simulink model "exampleModel_bus_axi_w_4ptavg"  (R2017b)
settings: Solver=VariableStepAuto  StartTime=0.0  StopTime=10e-5  RelTol=1e-3
PreLoadFcn:
  | setup
values from neighbouring files (symbols this model uses):
  axiClk = 156.25e6    (= 156250000)    [setup.m]    (also in setup_exampleModel_bus_axi_simulink.m; setup_exampleModel_bus_axi_simulink_lcls2.m; setup_lcls2_pcav.m; sysgen_signal.m)
  cav1p1_addr = 204    [setup_exampleModel_bus_axi_simulink.m]    (also in setup_exampleModel_bus_axi_simulink_lcls2.m; setup_lcls2_pcav.m; sysgen_signal.m)
  cav1p2_addr = cav1p1_addr * 2    (= 408)    [setup_exampleModel_bus_axi_simulink.m]    (also in setup_exampleModel_bus_axi_simulink_lcls2.m; setup_lcls2_pcav.m; sysgen_signal.m)
  cav2p1_addr = cav1p1_addr * 3    (= 612)    [setup_exampleModel_bus_axi_simulink.m]    (also in setup_exampleModel_bus_axi_simulink_lcls2.m; setup_lcls2_pcav.m; sysgen_signal.m)
  cav2p2_addr = cav1p1_addr * 4    (= 816)    [setup_exampleModel_bus_axi_simulink.m]    (also in setup_exampleModel_bus_axi_simulink_lcls2.m; setup_lcls2_pcav.m; sysgen_signal.m)
  Fadc = Fs/interleavedChannels    (= 29750000)    [setup.m]    (also in setup_exampleModel_bus_axi_simulink.m = 357000000; setup_exampleModel_bus_axi_simulink_lcls2.m = 351000000; setup_lcls2_pcav.m = 357000000; sysgen_signal.m = 357000000)
  fir_lpf = fir1(15, w_lpf)    [setup_exampleModel_bus_axi_simulink.m]    (also in setup_exampleModel_bus_axi_simulink_lcls2.m; setup_lcls2_pcav.m)
  Fproc = 204e6    (= 204000000)    [setup_exampleModel_bus_axi_simulink.m]    (also in setup_exampleModel_bus_axi_simulink_lcls2.m = 200571400; setup_lcls2_pcav.m; sysgen_signal.m)
  Fsig = Fproc/12    (= 17000000)    [setup_exampleModel_bus_axi_simulink.m]    (also in setup_exampleModel_bus_axi_simulink_lcls2.m = 16714283.3333; setup_lcls2_pcav.m)
  Tadc = 1/fadc    (= 2.80112044818e-09)    [cavity_signal.m]    (also in setup_exampleModel_bus_axi_simulink.m; setup_exampleModel_bus_axi_simulink_lcls2.m = 2.849002849e-09; setup_lcls2_pcav.m; setup_pcav_simulink.m)
undefined symbols (not defined in the file or in its folder): AXI4, Lite
libraries: xbsIndex_r4 x2870, llrf_lib x10, simulink x3
(part 6 of 15)

== system exampleModel_bus_axi_w_4ptavg/example/dsp/RFLib_input ==
  note: x12 time multiplex
  note: 204MHz clock domain, 12 interleaved channels = 17MHz/channel
  PA_in : Inport
  phaseAmpSync_in : Inport  Port=2
  chan_num : Inport  Port=3
  ddcSync_in : Inport  Port=4
  Bus Creator : BusCreator  Inputs=4
  Bus Creator1 : BusCreator  Inputs=4
  Complex to Magnitude-Angle : ComplexToMagnitudeAngle
  Complex to Real-Imag : ComplexToRealImag
  Register{25..31,34} (8 alike) : xbsIndex_r4/Register  init=0  rst=off  en=off  dbl_ovrd=off  block_type=register
  Unbuffer{,1..3} (4 alike) : Unbuffer
  amp : xbsIndex_r4/Gateway In  gui_display_data_type=Fixed-point  arith_type="Signed  (2's comp)"  n_bits=18  bin_pt=17  preci_type=Single  exp_width=8  frac_width=24  rows=1  columns=1  quantization="Round  (unbiased: +/- Inf)"  overflow=Saturate  period=1/Fproc  UseAsADC=off  ADCChannel='1'  interface=None  automatic_assignment=on  address_offset=hex2dec('00')  intf_name=''  intf_description=''  default_value=0  timing_constraint=None  locs_specified=off  LOCs={}  io_standard={}  inherit_from_input=off  hdl_port=on  dbl_ovrd=off  block_type=gatewayin
  ddcChannel : xbsIndex_r4/Gateway In  gui_display_data_type=Fixed-point  arith_type=Unsigned  n_bits=4  bin_pt=0  preci_type=Single  exp_width=8  frac_width=24  rows=1  columns=1  quantization="Round  (unbiased: +/- Inf)"  overflow=Saturate  period=1/Fproc  UseAsADC=off  ADCChannel='1'  interface=None  automatic_assignment=on  address_offset=hex2dec('00')  intf_name=''  intf_description=''  default_value=0  timing_constraint=None  locs_specified=off  LOCs={}  io_standard={}  inherit_from_input=off  hdl_port=on  dbl_ovrd=off  block_type=gatewayin
  ddcI : xbsIndex_r4/Gateway In  gui_display_data_type=Fixed-point  arith_type="Signed  (2's comp)"  n_bits=18  bin_pt=17  preci_type=Single  exp_width=8  frac_width=24  rows=1  columns=1  quantization="Round  (unbiased: +/- Inf)"  overflow=Saturate  period=1/Fproc  UseAsADC=off  ADCChannel='1'  interface=None  automatic_assignment=on  address_offset=hex2dec('00')  intf_name=''  intf_description=''  default_value=0  timing_constraint=None  locs_specified=off  LOCs={}  io_standard={}  inherit_from_input=off  hdl_port=on  dbl_ovrd=off  block_type=gatewayin
  ddcQ : xbsIndex_r4/Gateway In  gui_display_data_type=Fixed-point  arith_type="Signed  (2's comp)"  n_bits=18  bin_pt=17  preci_type=Single  exp_width=8  frac_width=24  rows=1  columns=1  quantization="Round  (unbiased: +/- Inf)"  overflow=Saturate  period=1/Fproc  UseAsADC=off  ADCChannel='1'  interface=None  automatic_assignment=on  address_offset=hex2dec('00')  intf_name=''  intf_description=''  default_value=0  timing_constraint=None  locs_specified=off  LOCs={}  io_standard={}  inherit_from_input=off  hdl_port=on  dbl_ovrd=off  block_type=gatewayin
  ddcSync : xbsIndex_r4/Gateway In  gui_display_data_type=Fixed-point  arith_type=Unsigned  n_bits=1  bin_pt=0  preci_type=Single  exp_width=8  frac_width=24  rows=1  columns=1  quantization="Round  (unbiased: +/- Inf)"  overflow=Saturate  period=1/Fproc  UseAsADC=off  ADCChannel='1'  interface=None  automatic_assignment=on  address_offset=hex2dec('00')  intf_name=''  intf_description=''  default_value=0  timing_constraint=None  locs_specified=off  LOCs={}  io_standard={}  inherit_from_input=off  hdl_port=on  dbl_ovrd=off  block_type=gatewayin
  phase : xbsIndex_r4/Gateway In  gui_display_data_type=Fixed-point  arith_type="Signed  (2's comp)"  n_bits=18  bin_pt=17  preci_type=Single  exp_width=8  frac_width=24  rows=1  columns=1  quantization="Round  (unbiased: +/- Inf)"  overflow=Saturate  period=1/Fproc  UseAsADC=off  ADCChannel='1'  interface=None  automatic_assignment=on  address_offset=hex2dec('00')  intf_name=''  intf_description=''  default_value=0  timing_constraint=None  locs_specified=off  LOCs={}  io_standard={}  inherit_from_input=off  hdl_port=on  dbl_ovrd=off  block_type=gatewayin
  phaseAmpChannel : xbsIndex_r4/Gateway In  gui_display_data_type=Fixed-point  arith_type=Unsigned  n_bits=4  bin_pt=0  preci_type=Single  exp_width=8  frac_width=24  rows=1  columns=1  quantization="Round  (unbiased: +/- Inf)"  overflow=Saturate  period=1/Fproc  UseAsADC=off  ADCChannel='1'  interface=None  automatic_assignment=on  address_offset=hex2dec('00')  intf_name=''  intf_description=''  default_value=0  timing_constraint=None  locs_specified=off  LOCs={}  io_standard={}  inherit_from_input=off  hdl_port=on  dbl_ovrd=off  block_type=gatewayin
  phaseAmpSync : xbsIndex_r4/Gateway In  gui_display_data_type=Fixed-point  arith_type=Unsigned  n_bits=1  bin_pt=0  preci_type=Single  exp_width=8  frac_width=24  rows=1  columns=1  quantization="Round  (unbiased: +/- Inf)"  overflow=Saturate  period=1/Fproc  UseAsADC=off  ADCChannel='1'  interface=None  automatic_assignment=on  address_offset=hex2dec('00')  intf_name=''  intf_description=''  default_value=0  timing_constraint=None  locs_specified=off  LOCs={}  io_standard={}  inherit_from_input=off  hdl_port=on  dbl_ovrd=off  block_type=gatewayin
  PA_out : Outport
  IQ_out : Outport  Port=2
  wires:
  phaseAmpSync_in/1 -> Unbuffer2/1
  amp/1 -> Register25/1
  phase/1 -> Register26/1
  phaseAmpChannel/1 -> Register27/1
  phaseAmpSync/1 -> Register28/1
  ddcI/1 -> Register29/1
  ddcQ/1 -> Register30/1
  ddcChannel/1 -> Register31/1
  PA_in/1 -> Unbuffer/1
  ddcSync/1 -> Register34/1
  Register25/1 -> Bus Creator/1  "amp"
  Register26/1 -> Bus Creator/2  "phase"
  Register27/1 -> Bus Creator/3  "channel"
  Register28/1 -> Bus Creator/4  "sync"
  Register29/1 -> Bus Creator1/1  "ddcI"
  Register30/1 -> Bus Creator1/2  "ddcQ"
  Register31/1 -> Bus Creator1/3  "ddcChannel"
  Register34/1 -> Bus Creator1/4  "ddcSync"
  chan_num/1 -> Unbuffer1/1
  Unbuffer1/1 -> phaseAmpChannel/1, ddcChannel/1
  Bus Creator/1 -> PA_out/1
  Unbuffer/1 -> Complex to Real-Imag/1, Complex to Magnitude-Angle/1
  Complex to Magnitude-Angle/1 -> amp/1
  Complex to Magnitude-Angle/2 -> phase/1
  Complex to Real-Imag/1 -> ddcI/1
  Complex to Real-Imag/2 -> ddcQ/1
  Bus Creator1/1 -> IQ_out/1
  ddcSync_in/1 -> Unbuffer3/1
  Unbuffer2/1 -> phaseAmpSync/1
  Unbuffer3/1 -> ddcSync/1

== system exampleModel_bus_axi_w_4ptavg/example/dsp/Ref ==
  In1 : Inport
  In2 : Inport  Port=2
  IQ_select : Subsystem
  PA_select : Subsystem
  Register3 : xbsIndex_r4/Register  init=0  rst=off  en=off  dbl_ovrd=off  block_type=register
  Register4 : xbsIndex_r4/Register  init=0  rst=off  en=off  dbl_ovrd=off  block_type=register
  Terminator : Terminator
  Terminator1 : Terminator
  ref_amp : Outport
  ref_phi : Outport  Port=2
  pa_sync : Outport  Port=3
  ref_i : Outport  Port=4
  ref_q : Outport  Port=5
  iq_sync : Outport  Port=6
  tag scope: rf_ref_amp=global, rf_ref_i=global, rf_ref_phase=global, rf_ref_q=global
  wires:
  In1/1 -> PA_select/1(PA_bus)
  In2/1 -> IQ_select/1(IQ_stream_in)
  IQ_select/3(sync) -> iq_sync/1
  PA_select/3(sync) -> pa_sync/1
  PA_select/1(Amp) -> [rf_ref_amp], ref_amp/1
  PA_select/2(Phase) -> [rf_ref_phase], ref_phi/1
  IQ_select/1(ddcI) -> [rf_ref_i], ref_i/1
  IQ_select/2(ddcQ) -> [rf_ref_q], ref_q/1
  [rf_ref_chan_sel] -> PA_select/2(PA_chan_sel)
  [rf_ref_chan_sel] -> IQ_select/2(IQ_chan_sel)
  [ref_window_start] -> Register3/1
  [ref_window_stop] -> Register4/1
  Register3/1 -> Terminator/1
  Register4/1 -> Terminator1/1

== system exampleModel_bus_axi_w_4ptavg/example/dsp/Subsystem1 ==
  input+noise : Inport
  CIC0 : DiscreteFir  Coefficients=ones(1,21)/21
  CIC1 : DiscreteFir  Coefficients=ones(1,21)/21
  CIC2 : DiscreteFir  Coefficients=ones(1,21)/21
  Downsample1 : DownSample  N=21  RateOptions=Allow multirate processing
  Gain : Gain  Gain=2/21
  Product : Product
  Real-Imag to Complex : RealImagToComplex
  cos : Sin  Frequency=2*pi*85e6  Phase=-pi/2  SampleTime=Tadc
  sin : Sin  Frequency=2*pi*85e6  SampleTime=Tadc
  complex : Outport
  wires:
  input+noise/1 -> Product/1
  Real-Imag to Complex/1 -> Gain/1
  cos/1 -> Real-Imag to Complex/1
  Gain/1 -> Product/2
  Product/1 -> CIC0/1
  sin/1 -> Real-Imag to Complex/2
  Downsample1/1 -> complex/1
  CIC2/1 -> Downsample1/1
  CIC0/1 -> CIC1/1
  CIC1/1 -> CIC2/1

== system exampleModel_bus_axi_w_4ptavg/example/dsp/Subsystem2 ==
  input+noise : Inport
  CIC0 : DiscreteFir  Coefficients=ones(1,21)/21
  CIC1 : DiscreteFir  Coefficients=ones(1,21)/21
  CIC2 : DiscreteFir  Coefficients=ones(1,21)/21
  Downsample1 : DownSample  N=21  RateOptions=Allow multirate processing
  Gain : Gain  Gain=2/21
  Product : Product
  Real-Imag to Complex : RealImagToComplex
  cos : Sin  Frequency=2*pi*85e6  Phase=-pi/2  SampleTime=Tadc
  sin : Sin  Frequency=2*pi*85e6  SampleTime=Tadc
  complex : Outport
  wires:
  CIC1/1 -> CIC2/1
  CIC0/1 -> CIC1/1
  CIC2/1 -> Downsample1/1
  Downsample1/1 -> complex/1
  sin/1 -> Real-Imag to Complex/2
  Product/1 -> CIC0/1
  Gain/1 -> Product/2
  cos/1 -> Real-Imag to Complex/1
  Real-Imag to Complex/1 -> Gain/1
  input+noise/1 -> Product/1

== system exampleModel_bus_axi_w_4ptavg/example/dsp/Cav1/DDC NCO1 ==
  Phase_ctrl : Inport
  Phase_reset : Inport  Port=2
  Bus Creator : BusCreator  Inputs=2
  Constant21 : xbsIndex_r4/Constant  const=1  gui_display_data_type=Boolean  arith_type=Boolean  n_bits=4  bin_pt=0  preci_type=Single  exp_width=8  frac_width=24  explicit_period=on  period=1/Fsig  equ=P=C  opselect=C  inp2=PCIN>>17  opr=+  inp1=P  carry=CIN  dbl_ovrd=off  block_type=constant
  Convert : xbsIndex_r4/Convert  gui_display_data_type=Boolean  arith_type=Boolean  n_bits=16  bin_pt=14  float_type=Single  exp_bits=8  fraction_bits=24  quantization=Truncate  overflow=Wrap  en=off  latency=1  pipeline=off  dbl_ovrd=off  block_type=convert
  "DDS Compiler 6.0 " : xbsIndex_r4/DDS Compiler 6.0   partspresent=Phase_Generator_and_SIN_COS_LUT  dds_clock_rate=17  channels=1  mode_of_operation=Standard  modulus=9  parameter_entry=Hardware_Parameters  spurious_free_dynamic_range=45  frequency_resolution=0.4  noise_shaping=Taylor_Series_Corrected  phase_width=32  output_width=26  output_selection=Sine_and_Cosine  negative_sine=off  negative_cosine=off  amplitude_mode=Unit_Circle  memory_type=Auto  optimization_goal=Auto  dsp48_use=Minimal  resync=on  latency_configuration=Auto  latency=1  has_phase_out=off  has_aclken=off  has_aresetn=off  explicit_period=off  period=1/Fproc  data_has_tlast=Not_Required  has_tready=on  s_phase_has_tuser=Not_Required  m_data_has_tuser=Not_Required  m_phase_has_tuser=Not_Required  s_phase_tuser_width=1  output_form=Twos_Complement  s_config_sync_mode=On_Vector  phase_increment=Streaming  output_frequency1=0  output_frequency2=0  output_frequency3=0  output_frequency4=0  output_frequency5=0  output_frequency6=0  output_frequency7=0  output_frequency8=0  output_frequency9=0  output_frequency10=0  output_frequency11=0  output_frequency12=0  output_frequency13=0  output_frequency14=0  output_frequency15=0  output_frequency16=0  pinc1='0'  pinc2='0'  pinc3='0'  pinc4='0'  pinc5='0'  pinc6='0'  pinc7='0'  pinc8='0'  pinc9='0'  pinc10='0'  pinc11='0'  pinc12='0'  pinc13='0'  pinc14='0'  pinc15='0'  pinc16='0'  phase_offset=None  phase_offset_angles1=0  phase_offset_angles2=0  phase_offset_angles3=0  phase_offset_angles4=0  phase_offset_angles5=0  phase_offset_angles6=0  phase_offset_angles7=0  phase_offset_angles8=0  phase_offset_angles9=0  phase_offset_angles10=0  phase_offset_angles11=0  phase_offset_angles12=0  phase_offset_angles13=0  phase_offset_angles14=0  phase_offset_angles15=0  phase_offset_angles16=0  poff1='0'  poff2='0'  poff3='0'  poff4='0'  poff5='0'  poff6='0'  poff7='0'  poff8='0'  poff9='0'  poff10='0'  poff11='0'  poff12='0'  poff13='0'  poff14='0'  poff15='0'  poff16='0'  trim_axipin_name=off  simulation_type=hybrid_sim  simulation_model=sysgen:xddsv6_0_cmodel  data_path_portlist={ 's_axis_config_tdata_poff', 's_axis_config_tdata_chan0_poff', 's_axis_config_tdata_pinc', 's_axis_config_tdata_chan0_pinc', 's_axis_phase_tdata_resync', 's_axis_phase_tdata_chan0_resync', 's_axis_phase_tdata_poff', 's_axis_phase_tdata_chan0_poff', 's_axis_phase_tdata_pinc', 's_axis_phase_tdata_chan0_pinc', 's_axis_phase_tdata_phase_in', 'm_axis_data_tdata_sine', 'm_axis_data_tdata_chan0_sine', 'm_axis_data_tdata_cosine', 'm_axis_data_tdata_chan0_cosine', 'm_axis_phase_tdata_phase_out', 'm_axis_phase_tdata_chan0_phase_out'}  por_mode=false  gui_behaviour=Sysgen  ip_name=DDS Compiler  ip_version=6.0  dsptool_ready=true  wrapper_available=true  port_translation_map={ 'aclken' => 'en', 'aresetn' => 'rst' }  ipcore_usecache=true  ipcore_useipmodelcache=true  ipcore_xco_need_fpga_part=true  ipcore_verbose=false  block_type=dds_compiler_v6_0
  Logical : xbsIndex_r4/Logical  logical_function=NAND  inputs=2  en=off  latency=1  precision=Full  arith_type=Unsigned  n_bits=16  bin_pt=0  align_bp=on  dbl_ovrd=off  block_type=logical
  pulse_catcher : Subsystem
  tvalid : Outport
  Out2 : Outport  Port=2
  Sine : Outport  Port=3
  Cosine : Outport  Port=4
  NCO_out : Outport  Port=5
  wires:
  "DDS Compiler 6.0 "/1 -> Out2/1
  Constant21/1 -> Logical/1
  Bus Creator/1 -> NCO_out/1
  "DDS Compiler 6.0 "/3 -> Bus Creator/1, Sine/1  "NCO_sin"
  "DDS Compiler 6.0 "/4 -> Bus Creator/2, Cosine/1  "NCO_cos"
  "DDS Compiler 6.0 "/2 -> tvalid/1
  Phase_reset/1 -> pulse_catcher/1(In1)
  Logical/1 -> "DDS Compiler 6.0 "/4, "DDS Compiler 6.0 "/1
  Convert/1 -> Logical/2
  pulse_catcher/1(Out1) -> "DDS Compiler 6.0 "/2, Convert/1
  Phase_ctrl/1 -> "DDS Compiler 6.0 "/3

== system exampleModel_bus_axi_w_4ptavg/example/dsp/Cav1/IQ_integration ==
  cav_windowed_imag : Inport
  cav_windowed_real : Inport  Port=2
  ref_windowed_i : Inport  Port=3
  ref_windowed_q : Inport  Port=4
  window_profile : Inport  Port=5
  Accumulator{,1..3} (4 alike) : xbsIndex_r4/Accumulator  operation=Add  n_bits=32  overflow=Wrap  scale=1  rst=on  hasbypass=off  infoeditControl=reset for floating point data type must be asserted for a minimum of 2 cycles  en=off  latency=1  msb_inp=100  msb=100  lsb=-100  use_behavioral_HDL=on  implementation=Fabric  dbl_ovrd=off  block_type=accum
  Convert{1,3,5..6} (4 alike) : xbsIndex_r4/Convert  gui_display_data_type=Boolean  arith_type=Boolean  n_bits=16  bin_pt=14  float_type=Single  exp_bits=8  fraction_bits=24  quantization=Truncate  overflow=Wrap  en=off  latency=1  pipeline=off  dbl_ovrd=off  block_type=convert
  Convert{2,4,9..10} (4 alike) : xbsIndex_r4/Convert  gui_display_data_type=Fixed-point  arith_type="Signed  (2's comp)"  n_bits=20  bin_pt=18  float_type=Single  exp_bits=8  fraction_bits=24  quantization=Truncate  overflow=Wrap  en=off  latency=1  pipeline=off  dbl_ovrd=off  block_type=convert
  Display{1..8} (8 alike) : Display
  Gateway Out{,1..18,22..23} (21 alike) : xbsIndex_r4/Gateway Out  inherit_from_input=off  hdl_port=on  rows=1  columns=1  UseAsDAC=off  DACChannel='1'  interface=None  automatic_assignment=on  address_offset=hex2dec('00')  intf_name=''  intf_description=''  timing_constraint=None  locs_specified=off  LOCs={}  io_standard={}  block_type=gatewayout
  Inverter{,1..3} (4 alike) : xbsIndex_r4/Inverter  en=off  latency=1  dbl_ovrd=off  block_type=inv
  Register{1..2,11..12} (4 alike) : xbsIndex_r4/Register  init=0  rst=off  en=on  dbl_ovrd=off  block_type=register
  Scope{1..9} (9 alike) : Scope  NumInputPorts=3
  cav_int_q : Outport
  cav_int_i : Outport  Port=2
  ref_int_i : Outport  Port=3
  ref_int_q : Outport  Port=4
  wires:
  Gateway Out13/1 -> Display2/1, Scope6/2
  Gateway Out6/1 -> Scope3/3, Scope7/3
  Accumulator1/1 -> Register11/1, Gateway Out7/1
  cav_windowed_real/1 -> Accumulator1/1, Gateway Out8/1
  Gateway Out/1 -> Scope6/3, Scope2/3
  Convert6/1 -> Register11/2, Inverter1/1
  [window] -> Convert5/1
  Convert5/1 -> Register12/2, Inverter/1
  Gateway Out8/1 -> Scope3/1, Scope7/1
  Accumulator/1 -> Register12/1, Gateway Out3/1
  Gateway Out9/1 -> Display1/1, Scope7/2
  Gateway Out3/1 -> Scope2/2
  Gateway Out5/1 -> Scope6/1, Scope2/1
  [window] -> Convert6/1
  Inverter/1 -> Gateway Out/1, Accumulator/2
  cav_windowed_imag/1 -> Gateway Out5/1, Accumulator/1
  Gateway Out7/1 -> Scope3/2
  Gateway Out23/1 -> Display4/1
  Gateway Out22/1 -> Display3/1
  Inverter1/1 -> Accumulator1/2, Gateway Out6/1
  Inverter2/1 -> Gateway Out2/1, Accumulator2/2
  Gateway Out1/1 -> Scope9/3, Display6/1
  Gateway Out4/1 -> Scope1/2
  [window] -> Convert1/1
  Gateway Out11/1 -> Scope9/1, Scope4/2, Display5/1
  Gateway Out10/1 -> Scope4/1, Scope1/1
  Convert1/1 -> Register1/2, Inverter2/1
  ref_windowed_i/1 -> Gateway Out10/1, Accumulator2/1
  Accumulator2/1 -> Gateway Out4/1, Register1/1
  Gateway Out2/1 -> Scope4/3, Scope1/3
  Gateway Out16/1 -> Scope5/3, Scope8/3
  Accumulator3/1 -> Register2/1, Gateway Out17/1
  ref_windowed_q/1 -> Accumulator3/1, Gateway Out14/1
  Convert3/1 -> Register2/2, Inverter3/1
  Gateway Out14/1 -> Scope5/1, Scope8/1
  Gateway Out15/1 -> Display7/1, Scope8/2
  [window] -> Convert3/1
  Gateway Out17/1 -> Scope5/2
  Gateway Out12/1 -> Display8/1
  Inverter3/1 -> Accumulator3/2, Gateway Out16/1
  Convert9/1 -> Gateway Out22/1, cav_int_i/1
  Convert10/1 -> cav_int_q/1, Gateway Out23/1
  Convert2/1 -> ref_int_i/1, Gateway Out1/1
  Convert4/1 -> ref_int_q/1, Gateway Out12/1
  window_profile/1 -> [window]
  Register1/1 -> Gateway Out18/1, Convert2/1, Gateway Out11/1
  Gateway Out18/1 -> Scope9/2
  Register2/1 -> Convert4/1, Gateway Out15/1
  Register11/1 -> Convert9/1, Gateway Out9/1
  Register12/1 -> Convert10/1, Gateway Out13/1

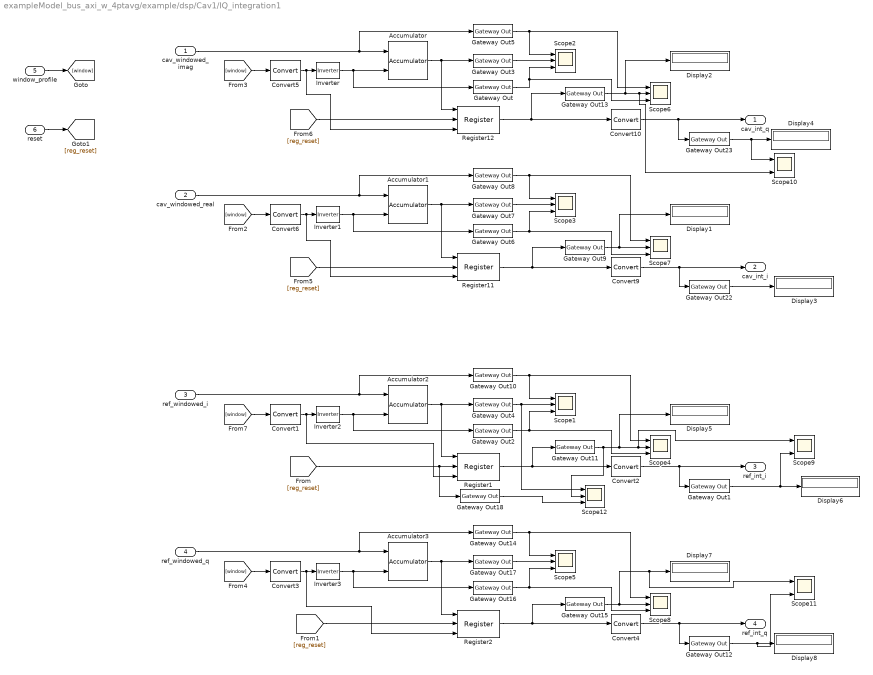
== system exampleModel_bus_axi_w_4ptavg/example/dsp/Cav1/IQ_integration1 ==
  cav_windowed_imag : Inport
  cav_windowed_real : Inport  Port=2
  ref_windowed_i : Inport  Port=3
  ref_windowed_q : Inport  Port=4
  window_profile : Inport  Port=5
  reset : Inport  Port=6
  Accumulator{,1..3} (4 alike) : xbsIndex_r4/Accumulator  operation=Add  n_bits=32  overflow=Wrap  scale=1  rst=on  hasbypass=off  infoeditControl=reset for floating point data type must be asserted for a minimum of 2 cycles  en=off  latency=1  msb_inp=100  msb=100  lsb=-100  use_behavioral_HDL=on  implementation=Fabric  dbl_ovrd=off  block_type=accum
  Convert{1,3,5..6} (4 alike) : xbsIndex_r4/Convert  gui_display_data_type=Boolean  arith_type=Boolean  n_bits=16  bin_pt=14  float_type=Single  exp_bits=8  fraction_bits=24  quantization=Truncate  overflow=Wrap  en=off  latency=1  pipeline=off  dbl_ovrd=off  block_type=convert
  Convert{2,4,9..10} (4 alike) : xbsIndex_r4/Convert  gui_display_data_type=Fixed-point  arith_type="Signed  (2's comp)"  n_bits=20  bin_pt=18  float_type=Single  exp_bits=8  fraction_bits=24  quantization=Truncate  overflow=Wrap  en=off  latency=1  pipeline=off  dbl_ovrd=off  block_type=convert
  Display{1..8} (8 alike) : Display
  Gateway Out{,1..18,22..23} (21 alike) : xbsIndex_r4/Gateway Out  inherit_from_input=off  hdl_port=on  rows=1  columns=1  UseAsDAC=off  DACChannel='1'  interface=None  automatic_assignment=on  address_offset=hex2dec('00')  intf_name=''  intf_description=''  timing_constraint=None  locs_specified=off  LOCs={}  io_standard={}  block_type=gatewayout
  Inverter{,1..3} (4 alike) : xbsIndex_r4/Inverter  en=off  latency=1  dbl_ovrd=off  block_type=inv
  Register{1..2,11..12} (4 alike) : xbsIndex_r4/Register  init=0  rst=on  en=on  dbl_ovrd=off  block_type=register
  Scope{1..12} (12 alike) : Scope  NumInputPorts=3
  cav_int_q : Outport
  cav_int_i : Outport  Port=2
  ref_int_i : Outport  Port=3
  ref_int_q : Outport  Port=4
  wires:
  Gateway Out13/1 -> Display2/1, Scope10/3, Scope6/2
  Gateway Out6/1 -> Scope3/3, Scope7/3
  Accumulator1/1 -> Register11/1, Gateway Out7/1
  cav_windowed_real/1 -> Accumulator1/1, Gateway Out8/1
  Gateway Out/1 -> Scope6/3, Scope2/3
  [window] -> Convert5/1
  Convert5/1 -> Register12/3, Inverter/1
  Gateway Out8/1 -> Scope3/1, Scope7/1
  Accumulator/1 -> Register12/1, Gateway Out3/1
  Gateway Out9/1 -> Display1/1, Scope7/2
  Gateway Out3/1 -> Scope2/2
  Gateway Out5/1 -> Scope6/1, Scope2/1
  [window] -> Convert6/1
  Inverter/1 -> Gateway Out/1, Accumulator/2
  cav_windowed_imag/1 -> Gateway Out5/1, Accumulator/1
  Gateway Out7/1 -> Scope3/2
  Gateway Out23/1 -> Scope10/1, Display4/1
  Gateway Out22/1 -> Display3/1
  Inverter1/1 -> Accumulator1/2, Gateway Out6/1
  Inverter2/1 -> Gateway Out2/1, Accumulator2/2
  Gateway Out1/1 -> Scope9/3, Display6/1
  Gateway Out4/1 -> Scope12/1, Scope1/2
  [window] -> Convert1/1
  Gateway Out11/1 -> Scope12/2, Scope9/1, Scope4/2, Display5/1
  Gateway Out10/1 -> Scope4/1, Scope1/1
  Convert1/1 -> Register1/3, Inverter2/1
  ref_windowed_i/1 -> Gateway Out10/1, Accumulator2/1
  Accumulator2/1 -> Gateway Out4/1, Register1/1
  Gateway Out2/1 -> Scope4/3, Scope1/3
  Gateway Out16/1 -> Scope5/3, Scope8/3
  Accumulator3/1 -> Register2/1, Gateway Out17/1
  ref_windowed_q/1 -> Accumulator3/1, Gateway Out14/1
  Gateway Out14/1 -> Scope5/1, Scope8/1
  Gateway Out15/1 -> Scope11/1, Display7/1, Scope8/2
  [window] -> Convert3/1
  Gateway Out17/1 -> Scope5/2
  Gateway Out12/1 -> Scope11/3, Display8/1
  Inverter3/1 -> Accumulator3/2, Gateway Out16/1
  Convert9/1 -> Gateway Out22/1, cav_int_i/1
  Convert10/1 -> cav_int_q/1, Gateway Out23/1
  Convert2/1 -> ref_int_i/1, Gateway Out1/1
  Convert4/1 -> ref_int_q/1, Gateway Out12/1
  window_profile/1 -> [window]
  Register1/1 -> Gateway Out11/1, Convert2/1
  Register2/1 -> Convert4/1, Gateway Out15/1
  Register11/1 -> Convert9/1, Gateway Out9/1
  Register12/1 -> Convert10/1, Gateway Out13/1
  reset/1 -> [reg_reset]
  [reg_reset] -> Gateway Out18/1, Register1/2
  Gateway Out18/1 -> Scope12/3
  Convert3/1 -> Register2/3, Inverter3/1
  [reg_reset] -> Register2/2
  [reg_reset] -> Register11/2
  Convert6/1 -> Register11/3, Inverter1/1
  [reg_reset] -> Register12/2

== system exampleModel_bus_axi_w_4ptavg/example/dsp/Cav1/Masking_n_delay ==
  note: delay for the comparison because Axilite register
      | takes a about 40 dsp clk cycles to load in
  phi_reset_trig : Inport
  start_pt : Inport  Port=2
  stop_pt : Inport  Port=3
  delay_amt : Inport  Port=4
  delay_latch : Inport  Port=5
  AddSub1 : xbsIndex_r4/AddSub  mode=Addition  use_carryin=off  use_carryout=off  en=off  latency=1  precision=User Defined  arith_type=Unsigned  n_bits=16  bin_pt=0  quantization=Truncate  overflow=Wrap  use_behavioral_HDL=off  hw_selection=Fabric  pipelined=off  dbl_ovrd=off  block_type=addsub
  AddSub4 : xbsIndex_r4/AddSub  mode=Addition  use_carryin=off  use_carryout=off  en=on  latency=1  precision=User Defined  arith_type=Unsigned  n_bits=16  bin_pt=0  quantization=Truncate  overflow=Saturate  use_behavioral_HDL=off  hw_selection=Fabric  pipelined=off  dbl_ovrd=off  block_type=addsub
  Constant1 : xbsIndex_r4/Constant  const=0  gui_display_data_type=Fixed-point  arith_type=Unsigned  n_bits=16  bin_pt=0  preci_type=Single  exp_width=8  frac_width=24  explicit_period=off  period=1  equ=P=C  opselect=C  inp2=PCIN>>17  opr=+  inp1=P  carry=CIN  dbl_ovrd=off  block_type=constant
  Constant11 : xbsIndex_r4/Constant  const=55  gui_display_data_type=Fixed-point  arith_type=Unsigned  n_bits=16  bin_pt=0  preci_type=Single  exp_width=8  frac_width=24  explicit_period=off  period=1  equ=P=C  opselect=C  inp2=PCIN>>17  opr=+  inp1=P  carry=CIN  dbl_ovrd=off  block_type=constant
  Constant2 : xbsIndex_r4/Constant  const=84  gui_display_data_type=Fixed-point  arith_type=Unsigned  n_bits=16  bin_pt=0  preci_type=Single  exp_width=8  frac_width=24  explicit_period=off  period=1  equ=P=C  opselect=C  inp2=PCIN>>17  opr=+  inp1=P  carry=CIN  dbl_ovrd=off  block_type=constant
  Constant3 : xbsIndex_r4/Constant  const=62  gui_display_data_type=Fixed-point  arith_type=Unsigned  n_bits=16  bin_pt=0  preci_type=Single  exp_width=8  frac_width=24  explicit_period=off  period=1  equ=P=C  opselect=C  inp2=PCIN>>17  opr=+  inp1=P  carry=CIN  dbl_ovrd=off  block_type=constant
  Constant4 : xbsIndex_r4/Constant  const=0  gui_display_data_type=Fixed-point  arith_type=Unsigned  n_bits=1  bin_pt=0  preci_type=Single  exp_width=8  frac_width=24  explicit_period=off  period=1  equ=P=C  opselect=C  inp2=PCIN>>17  opr=+  inp1=P  carry=CIN  dbl_ovrd=off  block_type=constant
  Convert1 : xbsIndex_r4/Convert  gui_display_data_type=Fixed-point  arith_type=Unsigned  n_bits=8  bin_pt=0  float_type=Single  exp_bits=8  fraction_bits=24  quantization=Truncate  overflow=Saturate  en=off  latency=1  pipeline=off  dbl_ovrd=off  block_type=convert
  Convert11 : xbsIndex_r4/Convert  gui_display_data_type=Fixed-point  arith_type=Unsigned  n_bits=1  bin_pt=0  float_type=Single  exp_bits=8  fraction_bits=24  quantization=Truncate  overflow=Wrap  en=off  latency=1  pipeline=off  dbl_ovrd=off  block_type=convert
  Convert2 : xbsIndex_r4/Convert  gui_display_data_type=Fixed-point  arith_type=Unsigned  n_bits=1  bin_pt=0  float_type=Single  exp_bits=8  fraction_bits=24  quantization=Truncate  overflow=Wrap  en=off  latency=1  pipeline=off  dbl_ovrd=off  block_type=convert
  Convert3 : xbsIndex_r4/Convert  gui_display_data_type=Boolean  arith_type=Boolean  n_bits=16  bin_pt=14  float_type=Single  exp_bits=8  fraction_bits=24  quantization=Truncate  overflow=Wrap  en=off  latency=1  pipeline=off  dbl_ovrd=off  block_type=convert
  Convert5 : xbsIndex_r4/Convert  gui_display_data_type=Boolean  arith_type=Boolean  n_bits=1  bin_pt=0  float_type=Single  exp_bits=8  fraction_bits=24  quantization=Truncate  overflow=Wrap  en=off  latency=1  pipeline=off  dbl_ovrd=off  block_type=convert
  Convert7 : xbsIndex_r4/Convert  gui_display_data_type=Boolean  arith_type=Boolean  n_bits=1  bin_pt=0  float_type=Single  exp_bits=8  fraction_bits=24  quantization=Truncate  overflow=Wrap  en=off  latency=1  pipeline=off  dbl_ovrd=off  block_type=convert
  Convert8 : xbsIndex_r4/Convert  gui_display_data_type=Boolean  arith_type=Boolean  n_bits=1  bin_pt=0  float_type=Single  exp_bits=8  fraction_bits=24  quantization=Truncate  overflow=Wrap  en=off  latency=1  pipeline=off  dbl_ovrd=off  block_type=convert
  Counter : xbsIndex_r4/Counter  cnt_type=Count Limited  cnt_to=2^15  operation=Up  start_count=0  cnt_by_val=1  arith_type=Unsigned  n_bits=16  bin_pt=0  load_pin=off  rst=on  en=on  explicit_period=on  period=12/Fproc  use_behavioral_HDL=off  implementation=Fabric  dbl_ovrd=off  block_type=counter
  Delay{,1..4,6..7} (7 alike) : xbsIndex_r4/Delay  rst=off  infoeditControl=Selection of Reset will increase slice count due to use of real FFs and instead of SRLs  en=off  latency=1  reg_retiming=off  dbl_ovrd=off  block_type=delay
  Delay8 : xbsIndex_r4/Delay  rst=off  infoeditControl=Selection of Reset will increase slice count due to use of real FFs and instead of SRLs  en=off  latency=4  reg_retiming=off  dbl_ovrd=off  block_type=delay
  Display1 : Display
  Down Sample1 : xbsIndex_r4/Down Sample  sample_ratio=12  sample_phase="Last Value of Frame  (most efficient)"  en=off  rst=off  latency=1  dbl_ovrd=off  block_type=dsamp
  Down Sample2 : xbsIndex_r4/Down Sample  sample_ratio=12  sample_phase="Last Value of Frame  (most efficient)"  en=off  rst=off  latency=1  dbl_ovrd=off  block_type=dsamp
  Gateway Out{4..11,27..29} (11 alike) : xbsIndex_r4/Gateway Out  inherit_from_input=off  hdl_port=on  rows=1  columns=1  UseAsDAC=off  DACChannel='1'  interface=None  automatic_assignment=on  address_offset=hex2dec('00')  intf_name=''  intf_description=''  timing_constraint=None  locs_specified=off  LOCs={}  io_standard={}  block_type=gatewayout
  Gateway Out16 : xbsIndex_r4/Gateway Out  inherit_from_input=off  hdl_port=off  rows=1  columns=1  UseAsDAC=off  DACChannel='1'  interface=None  automatic_assignment=on  address_offset=hex2dec('00')  intf_name=''  intf_description=''  timing_constraint=None  locs_specified=off  LOCs={}  io_standard={}  block_type=gatewayout
  Gateway Out17 : xbsIndex_r4/Gateway Out  inherit_from_input=off  hdl_port=off  rows=1  columns=1  UseAsDAC=off  DACChannel='1'  interface=None  automatic_assignment=on  address_offset=hex2dec('00')  intf_name=''  intf_description=''  timing_constraint=None  locs_specified=off  LOCs={}  io_standard={}  block_type=gatewayout
  Gateway Out18 : xbsIndex_r4/Gateway Out  inherit_from_input=off  hdl_port=off  rows=1  columns=1  UseAsDAC=off  DACChannel='1'  interface=None  automatic_assignment=on  address_offset=hex2dec('00')  intf_name=''  intf_description=''  timing_constraint=None  locs_specified=off  LOCs={}  io_standard={}  block_type=gatewayout
  Logical1 : xbsIndex_r4/Logical  logical_function=AND  inputs=2  en=off  latency=1  precision=Full  arith_type=Unsigned  n_bits=16  bin_pt=0  align_bp=on  dbl_ovrd=off  block_type=logical
  Logical2 : xbsIndex_r4/Logical  logical_function=AND  inputs=2  en=off  latency=1  precision=Full  arith_type=Unsigned  n_bits=16  bin_pt=0  align_bp=on  dbl_ovrd=off  block_type=logical
  Register : xbsIndex_r4/Register  init=49  rst=off  en=on  dbl_ovrd=off  block_type=register
  Register1 : xbsIndex_r4/Register  init=0  rst=off  en=on  dbl_ovrd=off  block_type=register
  Register10 : xbsIndex_r4/Register  init=0  rst=off  en=off  dbl_ovrd=off  block_type=register
  Register5 : xbsIndex_r4/Register  init=0  rst=off  en=off  dbl_ovrd=off  block_type=register
  Register6 : xbsIndex_r4/Register  init=100  rst=off  en=off  dbl_ovrd=off  block_type=register
  Relational1 : xbsIndex_r4/Relational  mode=a<b  op_type=Bool  en=on  latency=1  dbl_ovrd=off  block_type=relational
  Relational2 : xbsIndex_r4/Relational  mode=a>b  op_type=Bool  en=off  latency=1  dbl_ovrd=off  block_type=relational
  Relational3 : xbsIndex_r4/Relational  mode=a<b  op_type=Bool  en=on  latency=1  dbl_ovrd=off  block_type=relational
  Relational4 : xbsIndex_r4/Relational  mode=a>b  op_type=Bool  en=on  latency=1  dbl_ovrd=off  block_type=relational
  Relational5 : xbsIndex_r4/Relational  mode=a<b  op_type=Bool  en=on  latency=1  dbl_ovrd=off  block_type=relational
  Relational6 : xbsIndex_r4/Relational  mode=a>b  op_type=Bool  en=on  latency=1  dbl_ovrd=off  block_type=relational
  Relational7 : xbsIndex_r4/Relational  mode=a>b  op_type=Bool  en=off  latency=1  dbl_ovrd=off  block_type=relational
  Scope{3,5..6,10} (4 alike) : Scope  NumInputPorts=3
  Scope2 : Scope  NumInputPorts=2
  Scope4 : Scope  NumInputPorts=2
  trig_reset : Outport
  counter : Outport  Port=2
  eval_window : Outport  Port=3
  integral_trig : Outport  Port=4
  flo_window : Outport  Port=5
  Stream_valid : Outport  Port=6
  delay_val : Outport  Port=7
  wires:
  Gateway Out5/1 -> Scope2/2
  start_pt/1 -> Register5/1
  phi_reset_trig/1 -> Register10/1
  Register5/1 -> Down Sample1/1
  stop_pt/1 -> Register6/1
  Register6/1 -> Down Sample2/1
  Convert3/1 -> Register1/2, Register1/1, Gateway Out6/1, trig_reset/1, Counter/1
  Delay2/1 -> Gateway Out10/1, Relational4/2
  Delay3/1 -> AddSub1/1, Relational3/2
  Constant1/1 -> Relational2/2
  Relational3/1 -> Gateway Out28/1, Convert7/1
  Relational4/1 -> Gateway Out27/1, Convert8/1
  Gateway Out28/1 -> Scope10/2
  Gateway Out29/1 -> Scope2/1, Scope10/3
  Gateway Out27/1 -> Scope6/3, Scope10/1
  Logical1/1 -> Convert11/1
  Convert8/1 -> Logical1/1
  Convert7/1 -> Logical1/2
  Convert11/1 -> eval_window/1, Gateway Out29/1
  Convert5/1 -> integral_trig/1, Gateway Out5/1
  Relational5/1 -> Convert5/1
  Relational2/1 -> Relational6/3, Relational1/3, Relational5/3, Relational3/3, Relational4/3
  Counter/1 -> Convert1/1
  Constant11/1 -> AddSub1/2
  AddSub1/1 -> Relational5/2
  Down Sample1/1 -> Delay2/1
  Down Sample2/1 -> Delay3/1
  Delay1/1 -> Gateway Out11/1, Relational4/1
  Delay4/1 -> Relational3/1
  Delay7/1 -> Relational1/1
  Constant2/1 -> Relational1/2
  Logical2/1 -> Convert2/1
  Relational1/1 -> Logical2/2
  Convert2/1 -> Gateway Out8/1, flo_window/1
  Delay6/1 -> Relational6/1
  Constant3/1 -> Relational6/2
  Relational6/1 -> Logical2/1
  Constant4/1 -> Relational7/2
  Relational7/1 -> Stream_valid/1
  Gateway Out4/1 -> Scope3/2
  Gateway Out6/1 -> Scope3/1
  Register10/1 -> Convert3/1
  Register1/1 -> Counter/2, Gateway Out7/1
  Gateway Out7/1 -> Scope3/3
  Gateway Out16/1 -> Scope5/1, Display1/1
  delay_latch/1 -> Gateway Out18/1, Delay/1, AddSub4/3
  delay_amt/1 -> AddSub4/2, Gateway Out16/1
  AddSub4/1 -> Register/1
  Gateway Out17/1 -> Scope5/2
  Gateway Out18/1 -> Scope5/3
  Register/1 -> AddSub4/1, delay_val/1, Gateway Out17/1
  Delay/1 -> Register/2
  Gateway Out8/1 -> Scope4/2
  Gateway Out9/1 -> Scope4/1
  Delay8/1 -> Gateway Out9/1
  Gateway Out11/1 -> Scope6/1
  Gateway Out10/1 -> Scope6/2
  Convert1/1 -> Gateway Out4/1, Relational7/1, Delay8/1, counter/1, Delay1/1, Delay4/1, Relational2/1, Delay6/1, Delay7/1, Relational5/1

== system exampleModel_bus_axi_w_4ptavg/example/dsp/Cav1/PA_conversion2 ==
  cav_int_q : Inport
  cav_int_i : Inport  Port=2
  ref_int_q : Inport  Port=3
  ref_int_i : Inport  Port=4
  integration_trig : Inport  Port=5
  cal_coefficient : Inport  Port=6
  AddSub : xbsIndex_r4/AddSub  mode=Subtraction  use_carryin=off  use_carryout=off  en=off  latency=1  precision=User Defined  arith_type="Signed  (2's comp)"  n_bits=18  bin_pt=15  quantization=Truncate  overflow=Wrap  use_behavioral_HDL=off  hw_selection=Fabric  pipelined=off  dbl_ovrd=off  block_type=addsub
  AddSub1 : xbsIndex_r4/AddSub  mode=Addition  use_carryin=off  use_carryout=off  en=off  latency=1  precision=User Defined  arith_type="Signed  (2's comp)"  n_bits=18  bin_pt=15  quantization=Truncate  overflow=Wrap  use_behavioral_HDL=off  hw_selection=Fabric  pipelined=off  dbl_ovrd=off  block_type=addsub
  CORDIC 6.0 1 : xbsIndex_r4/CORDIC 6.0   functional_selection=Translate  architectural_configuration=Parallel  pipelining_mode=Maximum  data_format=SignedFraction  phase_format=Scaled_Radians  input_width=20  output_width=18  round_mode=Truncate  iterations=0  precision=0  compensation_scaling=No_Scale_Compensation  coarse_rotation=on  aclken=off  aresetn=off  out_tready=off  cartesian_has_tuser=off  cartesian_has_tlast=off  cartesian_tuser_width=1  phase_has_tuser=off  phase_has_tlast=off  phase_tuser_width=1  out_tlast_behv=Null  flow_control=NonBlocking  optimize_goal=Resources  trim_axipin_name=on  simulation_type=hybrid_sim  simulation_model=sysgen:cordic_v6_0  data_path_portlist={'s_axis_cartesian_tdata_imag', 's_axis_cartesian_tdata_real', 's_axis_phase_tdata_phase', 'm_axis_dout_tdata_imag', 'm_axis_dout_tdata_real', 'm_axis_dout_tdata_phase','m_axis_dout_tdata'}  ip_name=CORDIC  ip_version=6.0  dsptool_ready=true  ipcore_usecache=true  ipcore_useipmodelcache=true  wrapper_available=true  port_translation_map={ 'aclken' => 'en', 'aresetn' => 'rst' }  block_type=cordic_v6_0
      settings: infoedit=CORDIC 6.0
  CORDIC 6.0 2 : xbsIndex_r4/CORDIC 6.0   functional_selection=Translate  architectural_configuration=Parallel  pipelining_mode=Maximum  data_format=SignedFraction  phase_format=Scaled_Radians  input_width=20  output_width=18  round_mode=Truncate  iterations=0  precision=0  compensation_scaling=No_Scale_Compensation  coarse_rotation=on  aclken=off  aresetn=off  out_tready=off  cartesian_has_tuser=off  cartesian_has_tlast=off  cartesian_tuser_width=1  phase_has_tuser=off  phase_has_tlast=off  phase_tuser_width=1  out_tlast_behv=Null  flow_control=NonBlocking  optimize_goal=Resources  trim_axipin_name=on  simulation_type=hybrid_sim  simulation_model=sysgen:cordic_v6_0  data_path_portlist={'s_axis_cartesian_tdata_imag', 's_axis_cartesian_tdata_real', 's_axis_phase_tdata_phase', 'm_axis_dout_tdata_imag', 'm_axis_dout_tdata_real', 'm_axis_dout_tdata_phase','m_axis_dout_tdata'}  ip_name=CORDIC  ip_version=6.0  dsptool_ready=true  ipcore_usecache=true  ipcore_useipmodelcache=true  wrapper_available=true  port_translation_map={ 'aclken' => 'en', 'aresetn' => 'rst' }  block_type=cordic_v6_0
      settings: infoedit=CORDIC 6.0
  Delay{,1..3} (4 alike) : xbsIndex_r4/Delay  rst=off  infoeditControl=Selection of Reset will increase slice count due to use of real FFs and instead of SRLs  en=off  latency=1  reg_retiming=off  dbl_ovrd=off  block_type=delay
  Gateway Out{1..5,9,13,20..22,30..31,33} (13 alike) : xbsIndex_r4/Gateway Out  inherit_from_input=off  hdl_port=off  rows=1  columns=1  UseAsDAC=off  DACChannel='1'  interface=None  automatic_assignment=on  address_offset=hex2dec('00')  intf_name=''  intf_description=''  timing_constraint=None  locs_specified=off  LOCs={}  io_standard={}  block_type=gatewayout
  Gateway Out{6..8,24..26} (6 alike) : xbsIndex_r4/Gateway Out  inherit_from_input=off  hdl_port=on  rows=1  columns=1  UseAsDAC=off  DACChannel='1'  interface=None  automatic_assignment=on  address_offset=hex2dec('00')  intf_name=''  intf_description=''  timing_constraint=None  locs_specified=off  LOCs={}  io_standard={}  block_type=gatewayout
  Inverter{1..4} (4 alike) : xbsIndex_r4/Inverter  en=off  latency=1  dbl_ovrd=off  block_type=inv
  Register{11..14} (4 alike) : xbsIndex_r4/Register  init=0  rst=off  en=on  dbl_ovrd=off  block_type=register
  Scope{1..3,6,8,14..15} (7 alike) : Scope  NumInputPorts=3
  phi_diff : Outport
  ref_phi_out : Outport  Port=2
  ref_amp_out : Outport  Port=3
  cav_phi_out : Outport  Port=4
  cav_amp_out : Outport  Port=5
  wires:
  Register14/1 -> Gateway Out31/1, cav_amp_out/1
  Register13/1 -> Gateway Out33/1, cav_phi_out/1, [cav_phi_out]
  Register12/1 -> Gateway Out13/1, ref_amp_out/1
  Register11/1 -> Gateway Out22/1, ref_phi_out/1, [ref_phi_out]
  cal_coefficient/1 -> AddSub1/2
  [cav_phi_out] -> AddSub1/1
  AddSub1/1 -> AddSub/1, Gateway Out2/1
  integration_trig/1 -> [trig]
  [trig] -> CORDIC 6.0 2/1, Gateway Out6/1
  Gateway Out4/1 -> Scope1/3
  Gateway Out2/1 -> Scope1/2
  Gateway Out1/1 -> Scope1/1
  AddSub/1 -> phi_diff/1, Gateway Out1/1
  [ref_phi_out] -> Gateway Out4/1, AddSub/2
  Delay3/1 -> Register11/1
  Delay2/1 -> Register12/1
  Delay1/1 -> Register13/1
  Delay/1 -> Register14/1
  ref_int_q/1 -> CORDIC 6.0 2/2, Gateway Out7/1
  cav_int_i/1 -> CORDIC 6.0 1/3, Gateway Out26/1
  Gateway Out6/1 -> Scope6/1
  CORDIC 6.0 1/2 -> Gateway Out20/1, Delay1/1
  Gateway Out24/1 -> Scope8/1
  Gateway Out13/1 -> Scope3/2
  Gateway Out9/1 -> Scope3/3, Scope2/1
  Inverter4/1 -> Register12/2, Gateway Out9/1
  Gateway Out20/1 -> Scope14/2
  ref_int_i/1 -> CORDIC 6.0 2/3, Gateway Out8/1
  Gateway Out30/1 -> Scope14/1, Scope15/3
  Gateway Out31/1 -> Scope15/2
  cav_int_q/1 -> CORDIC 6.0 1/2, Gateway Out25/1
  Gateway Out3/1 -> Scope2/2
  Gateway Out21/1 -> Scope14/3
  Gateway Out5/1 -> Scope2/3
  [trig] -> CORDIC 6.0 1/1, Gateway Out24/1
  Inverter3/1 -> Register14/2, Gateway Out30/1
  CORDIC 6.0 2/2 -> Delay3/1, Gateway Out3/1
  Gateway Out26/1 -> Scope8/3
  Gateway Out25/1 -> Scope8/2
  CORDIC 6.0 1/3 -> Gateway Out21/1, Delay/1
  Inverter1/1 -> Register11/2
  Gateway Out22/1 -> Scope3/1
  Gateway Out7/1 -> Scope6/2
  Inverter2/1 -> Register13/2
  CORDIC 6.0 2/1 -> Inverter1/1, Inverter4/1
  Gateway Out33/1 -> Scope15/1
  CORDIC 6.0 1/1 -> Inverter3/1, Inverter2/1
  Gateway Out8/1 -> Scope6/3
  CORDIC 6.0 2/3 -> Delay2/1, Gateway Out5/1

== system exampleModel_bus_axi_w_4ptavg/example/dsp/Cav1/PA_select ==
  PA_bus : Inport
  PA_chan_sel : Inport  Port=2
  Bus Creator3 : BusCreator  Inputs=3
  Bus Selector : BusSelector  OutputSignals=amp,phase,sync
  Bus Selector1 : BusSelector  OutputSignals=amp,phase,sync,channel
  Channel Select1 : llrf_lib/Sysgen/Single Rate/Channel Select  SystemSampleTime=-1
      settings: SourceProductName=LLRF Library
  Amp : Outport
  Phase : Outport  Port=2
  sync : Outport  Port=3
  wires:
  Bus Selector/3 -> sync/1  "<sync>"
  Bus Selector/2 -> Phase/1  "<phase>"
  Bus Selector/1 -> Amp/1  "<amp>"
  Bus Selector1/1 -> Channel Select1/1  "<amp>"
  Bus Selector1/2 -> Channel Select1/2  "<phase>"
  Bus Selector1/3 -> Channel Select1/3  "<sync>"
  Bus Selector1/4 -> Channel Select1/4  "<channel>"
  Channel Select1/1 -> Bus Creator3/1  "amp"
  Channel Select1/2 -> Bus Creator3/2  "phase"
  Channel Select1/3 -> Bus Creator3/3  "sync"
  Bus Creator3/1 -> Bus Selector/1
  PA_chan_sel/1 -> Channel Select1/5
  PA_bus/1 -> Bus Selector1/1

== system exampleModel_bus_axi_w_4ptavg/example/dsp/Cav1/PA_select1 ==
  PA_bus : Inport
  PA_chan_sel : Inport  Port=2
  Bus Creator3 : BusCreator  Inputs=3
  Bus Selector : BusSelector  OutputSignals=amp,phase,sync
  Bus Selector1 : BusSelector  OutputSignals=amp,phase,sync,channel
  Channel Select1 : llrf_lib/Sysgen/Single Rate/Channel Select  SystemSampleTime=-1
      settings: SourceProductName=LLRF Library
  Amp : Outport
  Phase : Outport  Port=2
  sync : Outport  Port=3
  wires:
  PA_bus/1 -> Bus Selector1/1
  PA_chan_sel/1 -> Channel Select1/5
  Bus Creator3/1 -> Bus Selector/1
  Channel Select1/3 -> Bus Creator3/3  "sync"
  Channel Select1/2 -> Bus Creator3/2  "phase"
  Channel Select1/1 -> Bus Creator3/1  "amp"
  Bus Selector1/4 -> Channel Select1/4  "<channel>"
  Bus Selector1/3 -> Channel Select1/3  "<sync>"
  Bus Selector1/2 -> Channel Select1/2  "<phase>"
  Bus Selector1/1 -> Channel Select1/1  "<amp>"
  Bus Selector/1 -> Amp/1  "<amp>"
  Bus Selector/2 -> Phase/1  "<phase>"
  Bus Selector/3 -> sync/1  "<sync>"
